simulink model "SPWM_3Phase_Inverter"  (R2025a)
settings: Solver=VariableStepAuto  StartTime=0.0  StopTime=10.0  RelTol=1e-3
libraries: spsCurrentMeasurementLib x3, spsVoltageMeasurementLib x3, spsAsynchronousMachineSIUnitsLib x1, spsDCVoltageSourceLib x1, simulink x1, spsSeriesRLCBranchLib x1, spsUniversalBridgeLib x1, sps_lib x1
settings Model: Creator=Apoorv  LastModifiedBy=Apoorv

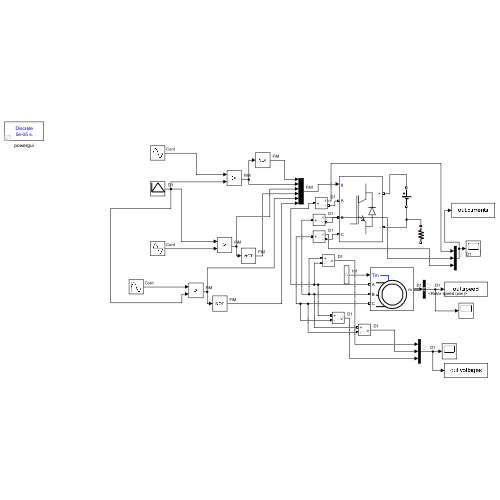
[thumbnail: Simulink's stored preview of the top-level diagram]
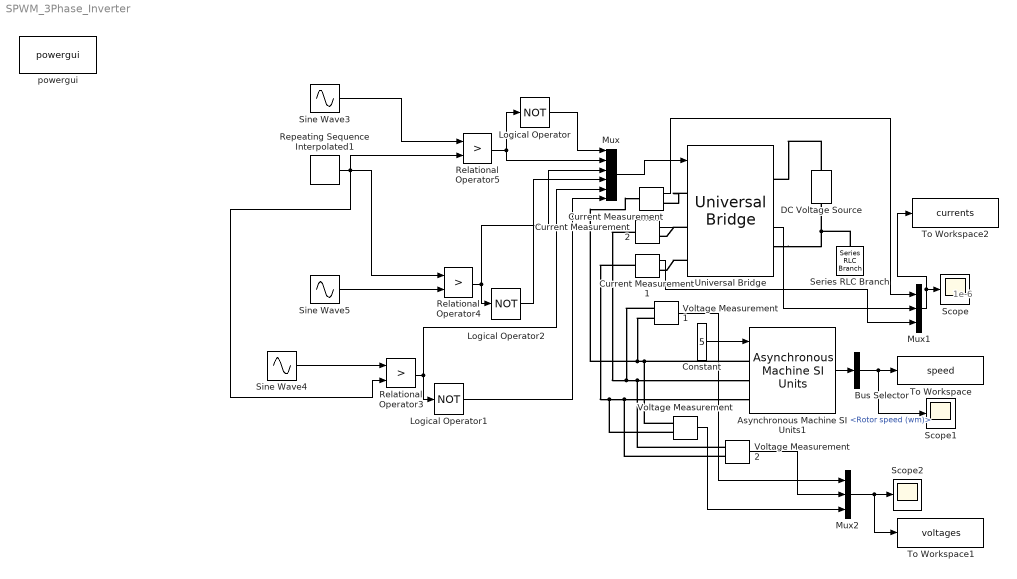
== system SPWM_3Phase_Inverter ==
  note: 1e-6
  Asynchronous Machine SI Units1 : spsAsynchronousMachineSIUnitsLib/Asynchronous Machine SI Units  RotorType=Squirrel-cage  PresetModel="02:  10 HP  460 V 60Hz 1760 RPM"  MechanicalLoad=Torque Tm  ShowDetailedParameters=on  ReferenceFrame=Rotor  Units=SI  MeasurementBus=off  NominalParameters=[7460 460 60]  VoltageRatio=1  Stator=[0.6837 0.004152]  Rotor=[0.451 0.004152]  Cage1=[0.4155 0.002066]  Cage2=[0.4168 0.0003495]  Lm=0.1486  Mechanical=[0.05 0.008141 2]  PolePairs=2  InitialConditions=[0 0 0 0 0 0 0 0]  SimulateSaturation=off  Saturation=[14.03593122, 27.81365428, 53.79336849, 72.68890987, 97.98006896, 148.6815601, 215.7428561, 302.9841135, 428.7778367 ; 230, 322, 414, 460, 506, 552, 598, 644, 690]  LoadFlowParameters=1492000  TsPowergui=0  TsBlock=-1  IterativeModel=Trapezoidal non iterative  IterativeDiscreteModel=Trapezoidal non iterative  Pmec=1.492e+006
  Bus Selector : BusSelector  OutputSignals=Mechanical.Rotor speed (wm)
  Constant : Constant  Value=5
  Current Measurement : spsCurrentMeasurementLib/Current Measurement  PhasorSimulation=off  OutputType=Complex  PSBequivalent=0
  Current Measurement1 : spsCurrentMeasurementLib/Current Measurement  PhasorSimulation=off  OutputType=Complex  PSBequivalent=0
  Current Measurement2 : spsCurrentMeasurementLib/Current Measurement  PhasorSimulation=off  OutputType=Complex  PSBequivalent=0
  DC Voltage Source : spsDCVoltageSourceLib/DC Voltage Source  Amplitude=100  Measurements=None
  Logical Operator : Logic  Operator=NOT  AllPortsSameDT=off  OutDataTypeStr=boolean
  Logical Operator1 : Logic  Operator=NOT  AllPortsSameDT=off  OutDataTypeStr=boolean
  Logical Operator2 : Logic  Operator=NOT  AllPortsSameDT=off  OutDataTypeStr=boolean
  Mux : Mux  Inputs=6
  Mux1 : Mux  Inputs=3
  Mux2 : Mux  Inputs=3
  Relational Operator3 : RelationalOperator  Operator=>  OutDataTypeStr=boolean  RndMeth=Simplest  InputSameDT=off
  Relational Operator4 : RelationalOperator  Operator=>  OutDataTypeStr=boolean  RndMeth=Simplest  InputSameDT=off
  Relational Operator5 : RelationalOperator  Operator=>  OutDataTypeStr=boolean  RndMeth=Simplest  InputSameDT=off
  Repeating Sequence Interpolated1 : simulink/Sources/Repeating Sequence Interpolated  OutValues=[0 1 0]  TimeValues=[0 0.0005 0.001]  LookUpMeth=Interpolation-Use End Values  tsamp=5e-5  OutMin=[]  OutMax=[]  OutDataTypeStr=double  OutputDataTypeScalingMode=double  OutDataType=fixdt(0,8)  OutScaling=2^-10
  Scope : Scope
      settings: ActiveDisplayYMinimum=-11.198403967716764  ActiveDisplayYMaximum=28.953464147051726
  Scope1 : Scope
      settings: ActiveDisplayYMinimum=-11.198403967716764  ActiveDisplayYMaximum=28.953464147051726
  Scope2 : Scope
      settings: ActiveDisplayYMinimum=-11.198403967716764  ActiveDisplayYMaximum=28.953464147051726  DataLoggingVariableName=ScopeData2
  Series RLC Branch : spsSeriesRLCBranchLib/Series RLC Branch  LConnTagsString=__new0  RConnTagsString=__new0  BranchType=R  Resistance=1e-6  Inductance=1e-3  SetiL0=off  InitialCurrent=0  Capacitance=1e-6  Setx0=off  InitialVoltage=0  Measurements=None
  Sine Wave3 : Sin  Tag=va  Frequency=50  Phase=-2*pi/3  SampleTime=0
  Sine Wave4 : Sin  Frequency=50  Phase=2*pi/3  SampleTime=0
  Sine Wave5 : Sin  Frequency=50  SampleTime=0
  To Workspace : ToWorkspace  VariableName=speed  SaveFormat=Timeseries  SampleTime=-1
  To Workspace1 : ToWorkspace  VariableName=voltages  SaveFormat=Timeseries  SampleTime=-1
  To Workspace2 : ToWorkspace  VariableName=currents  SaveFormat=Timeseries  SampleTime=-1
  Universal Bridge : spsUniversalBridgeLib/Universal Bridge  Arms=3  SnubberResistance=1e5  SnubberCapacitance=inf  Device=IGBT / Diodes  Ron=1e-3  Lon=0  ForwardVoltages="[  0  0  ]"  ForwardVoltage=0  GTOparameters=[ 10e-6 , 20e-6 ]  IGBTparameters=[ 1e-6 , 2e-6 ]  Measurements=All voltages and currents  Measurements_2=None  converterType=Rectifier
  Voltage Measurement : spsVoltageMeasurementLib/Voltage Measurement  PhasorSimulation=off  OutputType=Complex  PSBequivalent=0
  Voltage Measurement1 : spsVoltageMeasurementLib/Voltage Measurement  PhasorSimulation=off  OutputType=Complex  PSBequivalent=0
  Voltage Measurement2 : spsVoltageMeasurementLib/Voltage Measurement  PhasorSimulation=off  OutputType=Complex  PSBequivalent=0
  powergui : sps_lib/powergui  Priority=1  SimulationMode=Discrete  SampleTime=5e-5  frequency=60  Iterations=50  frequencyindice=60  Pbase=100e6  ErrMax=1e-4  UnitsV=kV  UnitsW=MW  buscounter=0  FunctionMessages=off  echomessages=off  EnableUseOfTLC=off  CurrentSourceSwitches=off  DisableSnubberDevices=off  DisableRonSwitches=off  DisableVfSwitches=off  DisplayEquations=off  AutomaticDiscreteSolvers=off  SolverType=Tustin/Backward Euler (TBE)  Interpol=off  ExternalGateDelay=off  methode=off  Ts=100  x0status=blocks  SPID=on  SwTol=0  HookPort=off  NonlinearTolerance=1e-4  nMaxIteration=100  ContinueOnMaxIteration=off  RestoreLinks=warning  ResistiveCurrentMeasurement=off  Frange=[0:2:500]  Ylog=off  Xlog=on  ShowGrid=off  save=off  variable=ZData  structure=0  ZoomFFT=off  StartTime=0.0  cycles=1  DisplayStyle=1  fundamental=60  FreqAxis=off  MaxFrequency=1000  frequencyindicesteady=1  RmsSteady=1  display=off
  wires:
  Sine Wave3/1 -> Relational Operator5/1
  Sine Wave4/1 -> Relational Operator3/1
  Sine Wave5/1 -> Relational Operator4/2
  Repeating Sequence Interpolated1/1 -> Relational Operator4/1, Relational Operator3/2, Relational Operator5/2
  Relational Operator5/1 -> Mux/2, Logical Operator/1
  Relational Operator4/1 -> Mux/3, Logical Operator2/1
  Relational Operator3/1 -> Mux/5, Logical Operator1/1
  Mux/1 -> Universal Bridge/1
  Logical Operator2/1 -> Mux/4
  Logical Operator1/1 -> Mux/6
  Logical Operator/1 -> Mux/1
  Constant/1 -> Asynchronous Machine SI Units1/1
  Current Measurement/1 -> Mux1/1
  Current Measurement2/1 -> Mux1/2
  Current Measurement1/1 -> Mux1/3
  Voltage Measurement/1 -> Mux2/3
  Mux1/1 -> Scope/1, To Workspace2/1
  Voltage Measurement1/1 -> Mux2/1
  Voltage Measurement2/1 -> Mux2/2
  Asynchronous Machine SI Units1/1 -> Bus Selector/1
  Bus Selector/1 -> Scope1/1, To Workspace/1  "<Rotor speed (wm)>"
  Mux2/1 -> To Workspace1/1, Scope2/1
  connections:
  Asynchronous Machine SI Units1/LConn1 -- Voltage Measurement/LConn1 -- Voltage Measurement1/LConn2 -- Current Measurement/LConn1
  Universal Bridge/LConn1 -- Current Measurement/RConn1
  Universal Bridge/LConn2 -- Current Measurement2/RConn1
  Current Measurement2/LConn1 -- Voltage Measurement1/LConn1 -- Voltage Measurement2/LConn1 -- Asynchronous Machine SI Units1/LConn2
  Universal Bridge/LConn3 -- Current Measurement1/RConn1
  Current Measurement1/LConn1 -- Voltage Measurement/LConn2 -- Voltage Measurement2/LConn2 -- Asynchronous Machine SI Units1/LConn3
  DC Voltage Source/RConn1 -- Universal Bridge/RConn1
  Universal Bridge/RConn2 -- Series RLC Branch/LConn1 -- DC Voltage Source/LConn1
